simulink model "Import_IMU"  (R2023b)
settings: Solver=FixedStepDiscrete  StartTime=0.0  StopTime=inf  FixedStep=0.003  RelTol=1e-3
InitFcn:
  | run('dual_leg_init.m');
values from neighbouring files (symbols this model uses):
  L1 = single(0.0804)    [dual_leg_init.m]
  L2 = single(0.1200)    [dual_leg_init.m]
  L3 = single(0.1200)    [dual_leg_init.m]
  L4 = single(0.0804)    [dual_leg_init.m]
  L5 = single(0.0700)    [dual_leg_init.m]
undefined symbols (not defined in the file or in its folder): CAL
libraries: ros2lib x14
(part 1 of 2)
settings Model: Creator=root  LastModifiedBy=root
settings OptimizationCC: EnhancedBackFolding=on  PassReuseOutputArgsAs=Individual arguments  ZeroExternalMemoryAtStartup=off  ZeroInternalMemoryAtStartup=off  MaxStackSize=64  OptimizeBlockOrder=speed  DifferentSizesBufferReuse=on  OptimizationCustomize=off  EfficientTunableParamExpr=on
settings DebuggingCC: ParameterTunabilityLossMsg=error
settings HardwareCC: ProdBitPerLong=64  ProdHWDeviceType=Intel->x86-64 (Linux 64)
settings SFSimCC: MATLABDynamicMemAlloc=off
settings RTWCC: Description=Embedded Coder  SystemTargetFile=ert.tlc  HardwareBoard=Robot Operating System 2 (ROS 2)  TLCOptions="-aInlineSetEventsForThisBaseRateFcn=TLC_FALSE -aSuppressMultiTaskScheduler=TLC_FALSE  -aRateBasedStepFcn=0"  TemplateMakefile=ert_default_tmf  Toolchain=Colcon Tools  TargetLang=C++
settings CodeAppCC: ForceParamTrailComments=on  IgnoreCustomStorageClasses=off  OperatorAnnotations=on  SimulinkDataObjDesc=on  SFDataObjDesc=on  InsertBlockDesc=on
settings ERTTargetCC: CodeInterfacePackaging=C++ class  SupportContinuousTime=on  RootIOFormat=Structure reference

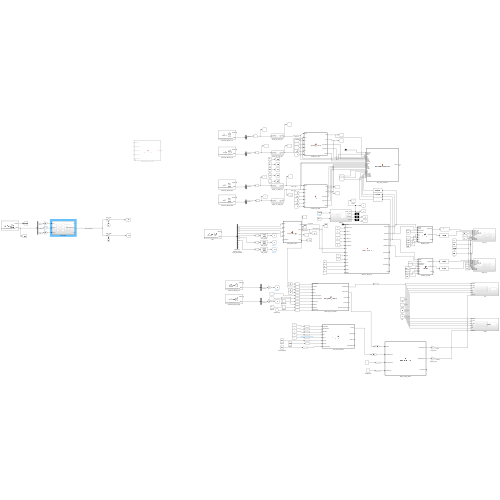
[thumbnail: Simulink's stored preview of the top-level diagram]
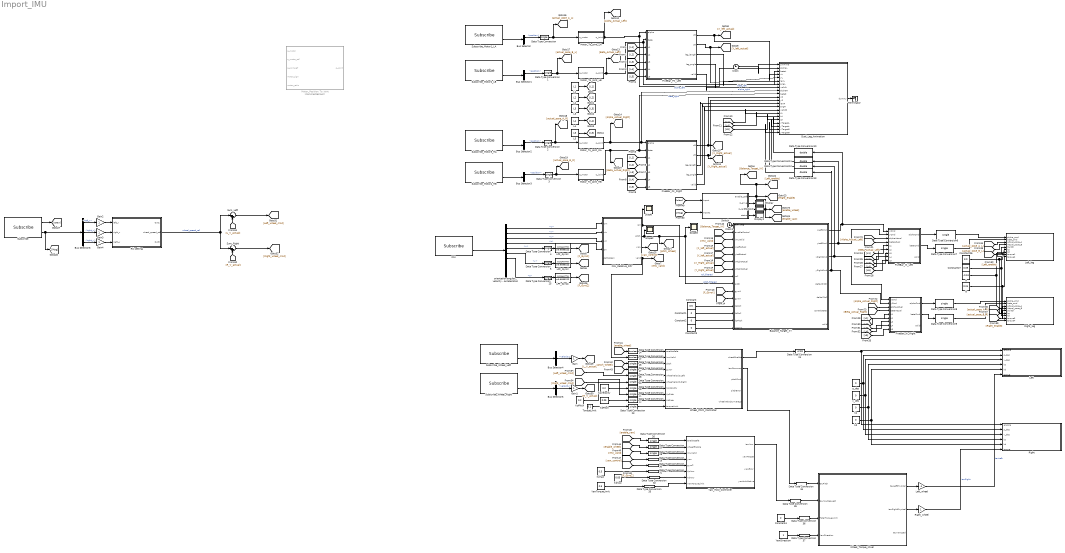
== system Import_IMU ==
  A : Constant  Value=-0.24
  B : Constant  Value=0.24
  Balance_Target_XY : MATLAB Function  TreatAsAtomicUnit=on
  Bus Selector{,1..5} (6 alike) : BusSelector  OutputSignals=position,velocity,torque
  Bus Selector6 : BusSelector  OutputSignals=left_x,right_x,right_y
  Clock : Clock
  Clock1 : Clock
  Constant : Constant  Value=0.5
  Constant1 : Constant  Value=0
  Constant2 : Constant  Value=0
  Constant26 : Constant  Value=3.0
  Constant27 : Constant  Value=0.09
  Constant3 : Constant  Value=0
  Constant4 : Constant  Value=2
  Data Type Conversion{,1..9,16..23,25..37} (31 alike) : DataTypeConversion  OutDataTypeStr=single  SaturateOnIntegerOverflow=off  RndMeth=Floor
  Data Type Conversion{10..13} (4 alike) : DataTypeConversion  OutDataTypeStr=double  SaturateOnIntegerOverflow=off  RndMeth=Floor
  Data Type Conversion14 : DataTypeConversion  OutDataTypeStr=boolean  SaturateOnIntegerOverflow=off  RndMeth=Floor
  Data Type Conversion15 : DataTypeConversion  OutDataTypeStr=boolean  SaturateOnIntegerOverflow=off  RndMeth=Floor
  Data Type Conversion24 : DataTypeConversion  OutDataTypeStr=uint8  SaturateOnIntegerOverflow=off  RndMeth=Floor
  Display : Display
  Display1 : Display
  Display2 : Display
  Dual_Leg_Animation : MATLAB Function  TreatAsAtomicUnit=on
  FiveBar_FK_Left : MATLAB Function  TreatAsAtomicUnit=on
  FiveBar_FK_Right : MATLAB Function  TreatAsAtomicUnit=on
  FiveBar_IK_Left : MATLAB Function  TreatAsAtomicUnit=on
  FiveBar_IK_Right : MATLAB Function  TreatAsAtomicUnit=on
  Gain : Gain
  Gain1 : Gain
  Gain2 : Gain  OutDataTypeStr=single
  Gain3 : Gain  OutDataTypeStr=single
  Gain4 : Gain  OutDataTypeStr=single
  IMU : ros2lib/Subscribe  topicSource=Select from ROS network  topic=/ecat/sn1966149/app1/read  messageType=sensor_msgs/Imu  sampleTime=-1  QOSHistory=Keep last  QOSDepth=1  QOSReliability=Best effort  QOSDurability=Volatile
  IMU_Relative_RPY : MATLAB Function  TreatAsAtomicUnit=on
  KdPitch : Constant  Value=0.05
  KdYaw : Constant  Value=0.05
  KpPitch : Constant  Value=0.2
  KpVelocity : Constant  Value=0.2
  KpYaw : Constant  Value=0.5
  L1 : Constant  Value=L1
  L2 : Constant  Value=L2
  L3 : Constant  Value=L3
  L4 : Constant  Value=L4
  L5 : Constant  Value=L5
  LPF_GyroX : DiscreteTransferFcn  Numerator=[0.3140778]  Denominator=[1 -0.6859222]
  LPF_GyroY : DiscreteTransferFcn  Numerator=[0.3140778]  Denominator=[1 -0.6859222]
  LPF_GyroZ : DiscreteTransferFcn  Numerator=[0.3140778]  Denominator=[1 -0.6859222]
  Left : Subsystem
  Left_leg : Subsystem
  Left_wheel : Gain  Gain=-1
  Motor_Position_To_Joint : MATLAB Function  Commented=on  TreatAsAtomicUnit=on
  Motor_To_Joint_LA : Subsystem
  Motor_To_Joint_LB : Subsystem
  Motor_To_Joint_RA : Subsystem
  Motor_To_Joint_RB : Subsystem
  RC setting : Subsystem
  Right : Subsystem
  Right_leg : Subsystem
  Right_wheel : Gain
  Scope : Scope
  Scope2 : Scope
  Scope3 : Scope
  Subscribe : ros2lib/Subscribe  topicSource=Select from ROS network  topic=/ecat/sn2228252/app1/read  messageType=custom_msgs/ReadDJIRC  sampleTime=-1  QOSHistory=Keep last  QOSDepth=1  QOSReliability=Best effort  QOSDurability=Volatile
  Subscribe_Motor1_LA : ros2lib/Subscribe  topicSource=Select from ROS network  topic=/ecat/sn2228252/app2/read  messageType=custom_msgs/ReadDmMotor  sampleTime=-1  QOSHistory=Keep last  QOSDepth=1  QOSReliability=Best effort  QOSDurability=Volatile
  Subscribe_Motor2_LB : ros2lib/Subscribe  topicSource=Select from ROS network  topic=/ecat/sn2228252/app3/read  messageType=custom_msgs/ReadDmMotor  sampleTime=-1  QOSHistory=Keep last  QOSDepth=1  QOSReliability=Best effort  QOSDurability=Volatile
  Subscribe_Motor3_RA : ros2lib/Subscribe  topicSource=Select from ROS network  topic=/ecat/sn2228252/app5/read  messageType=custom_msgs/ReadDmMotor  sampleTime=-1  QOSHistory=Keep last  QOSDepth=1  QOSReliability=Best effort  QOSDurability=Volatile
  Subscribe_Motor4_RB : ros2lib/Subscribe  topicSource=Select from ROS network  topic=/ecat/sn2228252/app6/read  messageType=custom_msgs/ReadDmMotor  sampleTime=-1  QOSHistory=Keep last  QOSDepth=1  QOSReliability=Best effort  QOSDurability=Volatile
  Subscribe_Wheel_Left : ros2lib/Subscribe  topicSource=Select from ROS network  topic=/ecat/sn2228252/app4/read  messageType=custom_msgs/ReadDmMotor  sampleTime=-1  QOSHistory=Keep last  QOSDepth=1  QOSReliability=Best effort  QOSDurability=Volatile
  Subscribe_Wheel_Right : ros2lib/Subscribe  topicSource=Select from ROS network  topic=/ecat/sn2228252/app7/read  messageType=custom_msgs/ReadDmMotor  sampleTime=-1  QOSHistory=Keep last  QOSDepth=1  QOSReliability=Best effort  QOSDurability=Volatile
  Sum_Left : Sum  Inputs=|-+
  Sum_Right : Sum  Inputs=|-+
  Switch : Subsystem
  Terminator : Terminator
  TorqueLimit : Constant  Value=0.1
  Wheel_Pitch_Controller : MATLAB Function  TreatAsAtomicUnit=on
  Wheel_Torque_Mixer : MATLAB Function  TreatAsAtomicUnit=on
  YawDirection : Constant
  YawTorqueLimit : Constant  Value=0.5
  Yaw_Hold_Controller : MATLAB Function  TreatAsAtomicUnit=on
  kd : Constant  Value=0  OutDataTypeStr=single
  kp : Constant  Value=0  OutDataTypeStr=single
  orientation angular_velocity linear_acceleration : BusSelector  OutputSignals=orientation.w,orientation.x,orientation.y,orientation.z,angular_velocity.x,angular_velocity.y,angular_velocity.z,linear_acceleration.x,linear_acceleration.y,linear_acceleration.z
  p_des : Constant  Value=0  OutDataTypeStr=single
  v_des : Constant  Value=0  OutDataTypeStr=single
  wires:
  Subscribe_Motor1_LA/2 -> Bus Selector/1
  Subscribe_Motor2_LB/2 -> Bus Selector1/1
  Subscribe_Motor3_RA/2 -> Bus Selector2/1
  Subscribe_Motor4_RB/2 -> Bus Selector3/1
  Bus Selector/1 -> Data Type Conversion/1  "<position>"
  Bus Selector1/1 -> Data Type Conversion1/1  "<position>"
  Bus Selector2/1 -> Data Type Conversion2/1  "<position>"
  Bus Selector3/1 -> Data Type Conversion3/1  "<position>"
  Motor_To_Joint_LA/1(q_joint) -> Dual_Leg_Animation/2(alphaL), FiveBar_FK_Left/1(alpha), [Alpha_Actual_Left]  "alpha_left"
  Motor_To_Joint_LB/1(q_joint) -> [Beta_Actual_Left], Dual_Leg_Animation/3(betaL), FiveBar_FK_Left/2(beta)  "beta_left"
  Motor_To_Joint_RA/1(q_joint) -> [Alpha_Actual_Right], Dual_Leg_Animation/9(alphaR), FiveBar_FK_Right/1(alpha)  "alpha_right"
  Motor_To_Joint_RB/1(q_joint) -> [Beta_Actual_Right], Dual_Leg_Animation/10(betaR), FiveBar_FK_Right/2(beta)  "beta_right"
  L1/1 -> [L1]
  L2/1 -> [L2]
  L3/1 -> [L3]
  L4/1 -> [L4]
  L5/1 -> [L5]
  [L1] -> FiveBar_FK_Left/3(L1)
  [L2] -> FiveBar_FK_Left/4(L2)
  [L3] -> FiveBar_FK_Left/5(L3)
  [L4] -> FiveBar_FK_Left/6(L4)
  [L5] -> FiveBar_FK_Left/7(L5)
  [L1] -> FiveBar_FK_Right/3(L1)
  [L2] -> FiveBar_FK_Right/4(L2)
  [L3] -> FiveBar_FK_Right/5(L3)
  [L4] -> FiveBar_FK_Right/6(L4)
  [L5] -> FiveBar_FK_Right/7(L5)
  Data Type Conversion/1 -> [actual_pose_A_L], Motor_To_Joint_LA/1(q_motor)
  Data Type Conversion1/1 -> [actual_pose_B_L], Motor_To_Joint_LB/1(q_motor)
  Data Type Conversion2/1 -> [actual_pose_A_R], Motor_To_Joint_RA/1(q_motor)
  Data Type Conversion3/1 -> [actual_pose_B_R], Motor_To_Joint_RB/1(q_motor)
  Clock/1 -> Dual_Leg_Animation/1(simTime)
  FiveBar_FK_Left/1(xB) -> [X_left_actual], Dual_Leg_Animation/4(xL)
  FiveBar_FK_Left/2(yB) -> [Y_left_actual], Dual_Leg_Animation/5(yL)
  FiveBar_FK_Left/3(leg_length) -> Dual_Leg_Animation/6(lenL)
  FiveBar_FK_Left/4(leg_angle) -> Dual_Leg_Animation/7(angL)
  FiveBar_FK_Left/5(valid) -> Dual_Leg_Animation/8(validL)
  FiveBar_FK_Right/1(xB) -> Dual_Leg_Animation/11(xR), [X_Right_actual]
  FiveBar_FK_Right/2(yB) -> [Y_Right_actual], Dual_Leg_Animation/12(yR)
  FiveBar_FK_Right/3(leg_length) -> Dual_Leg_Animation/13(lenR)
  FiveBar_FK_Right/4(leg_angle) -> Dual_Leg_Animation/14(angR)
  FiveBar_FK_Right/5(valid) -> Dual_Leg_Animation/15(validR)
  [L1] -> Dual_Leg_Animation/16(L1)
  [L4] -> Dual_Leg_Animation/17(L4)
  [L5] -> Dual_Leg_Animation/18(L5)
  Dual_Leg_Animation/1(dummy) -> Terminator/1
  IMU/2 -> orientation angular_velocity linear_acceleration/1
  orientation angular_velocity linear_acceleration/1 -> IMU_Relative_RPY/1(wIn)  "<w>"
  orientation angular_velocity linear_acceleration/2 -> IMU_Relative_RPY/2(xIn)  "<x>"
  orientation angular_velocity linear_acceleration/3 -> IMU_Relative_RPY/3(yIn)  "<y>"
  orientation angular_velocity linear_acceleration/4 -> IMU_Relative_RPY/4(zIn)  "<z>"
  IMU_Relative_RPY/1(roll) -> Balance_Target_XY/8(roll), Scope/1  "roll_filtered"
  IMU_Relative_RPY/2(pitch) -> [pitch_Wheel], Scope3/1, Balance_Target_XY/9(pitch), Scope2/1  "pitch_filtered"
  orientation angular_velocity linear_acceleration/5 -> Data Type Conversion4/1  "<x>"
  orientation angular_velocity linear_acceleration/6 -> Data Type Conversion5/1  "<y>"
  Data Type Conversion4/1 -> LPF_GyroX/1
  Data Type Conversion5/1 -> LPF_GyroY/1
  LPF_GyroX/1 -> [F_GyroX]
  LPF_GyroY/1 -> [F_GyroY]
  [F_GyroX] -> Balance_Target_XY/10(gyroX)
  [F_GyroY] -> Balance_Target_XY/11(gyroY)
  Clock1/1 -> Balance_Target_XY/1(simTime)
  [IMU_valid] -> Balance_Target_XY/3(imuValid)
  [X_left_actual] -> Balance_Target_XY/4(xLeftActual)
  [Y_left_actual] -> Balance_Target_XY/5(yLeftActual)
  [X_Right_actual] -> Balance_Target_XY/6(xRightActual)
  [Y_Right_actual] -> Balance_Target_XY/7(yRightActual)
  Constant/1 -> Balance_Target_XY/12(kpRoll)
  Constant1/1 -> Balance_Target_XY/13(kdRoll)
  Constant2/1 -> Balance_Target_XY/14(kpPitch)
  Constant3/1 -> Balance_Target_XY/15(kdPitch)
  Balance_Target_XY/1(xLeftCmd) -> Data Type Conversion10/1, FiveBar_IK_Left/1(xCmd)
  Balance_Target_XY/2(yLeftCmd) -> Data Type Conversion11/1, FiveBar_IK_Left/2(yCmd)
  Balance_Target_XY/3(xRightCmd) -> Data Type Conversion12/1, FiveBar_IK_Right/1(xCmd)
  Balance_Target_XY/4(yRightCmd) -> FiveBar_IK_Right/2(yCmd), Data Type Conversion13/1
  [Alpha_Actual_Left] -> FiveBar_IK_Left/3(alphaActual)
  [Beta_Actual_Left] -> FiveBar_IK_Left/4(betaActual)
  [Alpha_Actual_Right] -> FiveBar_IK_Right/3(alphaActual)
  [Beta_Actual_Right] -> FiveBar_IK_Right/4(betaActual)
  [L1] -> FiveBar_IK_Left/5(L1)
  [L2] -> FiveBar_IK_Left/6(L2)
  [L3] -> FiveBar_IK_Left/7(L3)
  [L4] -> FiveBar_IK_Left/8(L4)
  [L5] -> FiveBar_IK_Left/9(L5)
  [L1] -> FiveBar_IK_Right/5(L1)
  [L2] -> FiveBar_IK_Right/6(L2)
  [L3] -> FiveBar_IK_Right/7(L3)
  [L4] -> FiveBar_IK_Right/8(L4)
  [L5] -> FiveBar_IK_Right/9(L5)
  IMU_Relative_RPY/4(valid) -> [IMU_valid], Data Type Conversion15/1
  FiveBar_IK_Left/1(alphaCmd) -> Data Type Conversion6/1
  Data Type Conversion6/1 -> Left_leg/1(alpha_cmd)
  FiveBar_IK_Left/2(betaCmd) -> Data Type Conversion7/1
  Data Type Conversion7/1 -> Left_leg/2(beta_cmd)
  FiveBar_IK_Right/1(alphaCmd) -> Data Type Conversion8/1
  Data Type Conversion8/1 -> Right_leg/1(alpha_cmd)
  FiveBar_IK_Right/2(betaCmd) -> Data Type Conversion9/1
  Data Type Conversion9/1 -> Right_leg/2(beta_cmd)
  [actual_pose_A_L] -> Left_leg/3(Actual_pose_A)
  [actual_pose_B_L] -> Left_leg/4(Actual_pose_B)
  [actual_pose_A_R] -> Right_leg/3(Actual_pose_A)
  [actual_pose_B_R] -> Right_leg/4(Actual_pose_B)
  [Right_enable] -> Right_leg/5(Switch)
  [Left_enable] -> Left_leg/5(Switch)
  Switch/1(enable_safe) -> [enable_yaw], [enable_wheel], [Right_enable], [Left_enable], [Balance_Target_XY]
  [Balance_Target_XY] -> Balance_Target_XY/2(enableControl)
  Switch/2(rc_alive) -> Display/1
  Switch/3(rc_ready) -> Display1/1
  Switch/4(status) -> Display2/1
  Constant26/1 -> Right_leg/6(kp), Left_leg/6(kp)
  Constant27/1 -> Right_leg/7(kd), Left_leg/7(kd)
  A/1 -> Left_leg/8(torque1), Right_leg/9(torque4)
  B/1 -> Right_leg/8(torque3), Left_leg/9(torque2)
  Data Type Conversion10/1 -> Dual_Leg_Animation/19(xTargetL)
  Data Type Conversion11/1 -> Dual_Leg_Animation/20(yTargetL)
  Data Type Conversion12/1 -> Dual_Leg_Animation/21(xTargetR)
  Data Type Conversion13/1 -> Dual_Leg_Animation/22(yTargetR)
  Subscribe_Wheel_Left/2 -> Bus Selector4/1
  Subscribe_Wheel_Right/2 -> Bus Selector5/1
  Bus Selector4/2 -> Gain/1  "<velocity>"
  Bus Selector5/2 -> Gain1/1  "<velocity>"
  Data Type Conversion14/1 -> Wheel_Pitch_Controller/1(enableSafe)
  Data Type Conversion15/1 -> Wheel_Pitch_Controller/2(imuValid)
  Data Type Conversion16/1 -> Wheel_Pitch_Controller/3(pitch)
  Data Type Conversion17/1 -> Wheel_Pitch_Controller/4(gyroY)
  Data Type Conversion18/1 -> Wheel_Pitch_Controller/5(wheelVelocityLeft)
  Data Type Conversion20/1 -> Wheel_Pitch_Controller/6(wheelVelocityRight)
  Data Type Conversion19/1 -> Wheel_Pitch_Controller/7(KpVelocity)
  Data Type Conversion21/1 -> Wheel_Pitch_Controller/8(KpPitch)
  Data Type Conversion22/1 -> Wheel_Pitch_Controller/9(KdPitch)
  Data Type Conversion23/1 -> Wheel_Pitch_Controller/10(torqueLimit)
  [enable_wheel] -> Data Type Conversion14/1
  [pitch_Wheel] -> Data Type Conversion16/1
  [F_GyroY] -> Data Type Conversion17/1
  KpVelocity/1 -> Data Type Conversion19/1
  KpPitch/1 -> Data Type Conversion21/1
  KdPitch/1 -> Data Type Conversion22/1
  TorqueLimit/1 -> Data Type Conversion23/1
  Wheel_Pitch_Controller/2(tauCommon) -> Data Type Conversion34/1
  Wheel_Pitch_Controller/1(wheelEnable) -> Data Type Conversion24/1
  Data Type Conversion24/1 -> Right/1(enable), Left/1(enable)
  p_des/1 -> Right/2(p_des), Left/2(p_des)
  v_des/1 -> Left/3(v_des), Right/3(v_des)
  kp/1 -> Right/4(kp), Left/4(kp)
  kd/1 -> Right/5(kd), Left/5(kd)
  orientation angular_velocity linear_acceleration/7 -> Data Type Conversion25/1  "<z>"
  Data Type Conversion25/1 -> LPF_GyroZ/1
  [enable_wheel] -> Data Type Conversion27/1
  [enable_yaw] -> Data Type Conversion26/1
  [IMU_valid] -> Data Type Conversion28/1
  IMU_Relative_RPY/3(yaw) -> [yaw_control]
  [yaw_control] -> Data Type Conversion29/1
  LPF_GyroZ/1 -> [F_GyroZ]
  [F_GyroZ] -> Data Type Conversion30/1
  YawTorqueLimit/1 -> Data Type Conversion33/1
  KdYaw/1 -> Data Type Conversion32/1
  KpYaw/1 -> Data Type Conversion31/1
  YawDirection/1 -> Data Type Conversion37/1
  Yaw_Hold_Controller/1(tauYaw) -> Data Type Conversion35/1
  Wheel_Torque_Mixer/1(tauLeftPhysical) -> Left_wheel/1
  Left_wheel/1 -> Left/6(torque)  "tauLeft"
  Wheel_Torque_Mixer/2(tauRightPhysical) -> Right_wheel/1
  Right_wheel/1 -> Right/6(torque)  "tauRight"
  Constant4/1 -> Data Type Conversion36/1
  Data Type Conversion26/1 -> Yaw_Hold_Controller/1(enableSafe)
  Data Type Conversion27/1 -> Yaw_Hold_Controller/2(wheelEnable)
  Data Type Conversion28/1 -> Yaw_Hold_Controller/3(imuValid)
  Data Type Conversion29/1 -> Yaw_Hold_Controller/4(yaw)
  Data Type Conversion30/1 -> Yaw_Hold_Controller/5(gyroZ)
  Data Type Conversion31/1 -> Yaw_Hold_Controller/6(KpYaw)
  Data Type Conversion32/1 -> Yaw_Hold_Controller/7(KdYaw)
  Data Type Conversion33/1 -> Yaw_Hold_Controller/8(YawTorqueLimit)
  Data Type Conversion34/1 -> Wheel_Torque_Mixer/1(tauPitch)
  Data Type Conversion35/1 -> Wheel_Torque_Mixer/2(tauYawRequest)
  Data Type Conversion36/1 -> Wheel_Torque_Mixer/3(TotalTorqueLimit)
  Data Type Conversion37/1 -> Wheel_Torque_Mixer/4(YawDirection)
  Subscribe/1 -> [IsNew]
  Subscribe/2 -> [Msg], Bus Selector6/1
  [IsNew] -> Switch/1(Inport)
  [Msg] -> Switch/2(Inport1)
  Bus Selector6/1 -> Gain2/1  "<left_x>"
  Bus Selector6/2 -> Gain3/1  "<right_x>"
  Bus Selector6/3 -> Gain4/1  "<right_y>"
  Gain3/1 -> RC setting/2(right_x)
  Gain2/1 -> RC setting/1(left_x)
  Gain4/1 -> RC setting/3(right_y)
  RC setting/2(wheel_speed_ref) -> Sum_Right/1, Sum_Left/1  "wheel_speed_ref"
  Gain/1 -> [L_V_actual]
  Gain1/1 -> [R_V_actual]
  [L_V_actual] -> Sum_Left/2
  [R_V_actual] -> Sum_Right/2
  Sum_Left/1 -> [Left_wheel_cmd]
  Sum_Right/1 -> [Right_wheel_cmd]
  [Left_wheel_cmd] -> Data Type Conversion18/1
  [Right_wheel_cmd] -> Data Type Conversion20/1

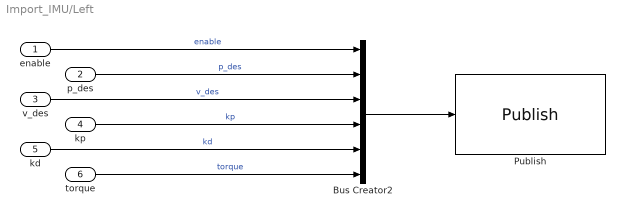
== system Import_IMU/Left ==
  enable : Inport
  p_des : Inport  Port=2
  v_des : Inport  Port=3
  kp : Inport  Port=4
  kd : Inport  Port=5
  torque : Inport  Port=6
  Bus Creator2 : BusCreator  Inputs=6  OutDataTypeStr=Bus: SL_Bus_custom_msgs_WriteDmMotorMITControl  NonVirtualBus=on
  Publish : ros2lib/Publish  topicSource=Select from ROS network  topic=/ecat/sn2228252/app4/write  messageType=custom_msgs/WriteDmMotorMITControl  QOSHistory=Keep last  QOSDepth=1  QOSReliability=Best effort  QOSDurability=Volatile
  wires:
  enable/1 -> Bus Creator2/1  "enable"
  Bus Creator2/1 -> Publish/1
  p_des/1 -> Bus Creator2/2  "p_des"
  v_des/1 -> Bus Creator2/3  "v_des"
  kp/1 -> Bus Creator2/4  "kp"
  kd/1 -> Bus Creator2/5  "kd"
  torque/1 -> Bus Creator2/6  "torque"

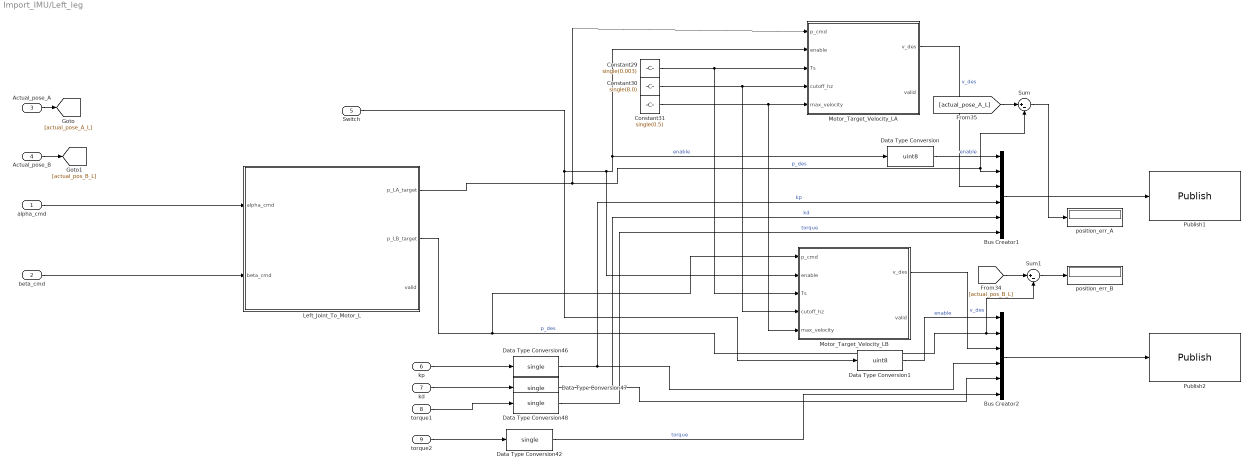
== system Import_IMU/Left_leg ==
  alpha_cmd : Inport
  beta_cmd : Inport  Port=2
  Actual_pose_A : Inport  Port=3
  Actual_pose_B : Inport  Port=4
  Switch : Inport  Port=5
  kp : Inport  Port=6
  kd : Inport  Port=7
  torque1 : Inport  Port=8
  torque2 : Inport  Port=9
  Bus Creator1 : BusCreator  Inputs=6  OutDataTypeStr=Bus: SL_Bus_custom_msgs_WriteDmMotorMITControl  NonVirtualBus=on
  Bus Creator2 : BusCreator  Inputs=6  OutDataTypeStr=Bus: SL_Bus_custom_msgs_WriteDmMotorMITControl  NonVirtualBus=on
  Constant29 : Constant  Value=single(0.003)
  Constant30 : Constant  Value=single(8.0)
  Constant31 : Constant  Value=single(0.5)
  Data Type Conversion : DataTypeConversion  OutDataTypeStr=uint8  SaturateOnIntegerOverflow=off  RndMeth=Floor
  Data Type Conversion1 : DataTypeConversion  OutDataTypeStr=uint8  SaturateOnIntegerOverflow=off  RndMeth=Floor
  Data Type Conversion{42,46..48} (4 alike) : DataTypeConversion  OutDataTypeStr=single  SaturateOnIntegerOverflow=off  RndMeth=Floor
  Left_Joint_To_Motor_L : MATLAB Function  TreatAsAtomicUnit=on
  Motor_Target_Velocity_LA : MATLAB Function  TreatAsAtomicUnit=on
  Motor_Target_Velocity_LB : MATLAB Function  TreatAsAtomicUnit=on
  Publish1 : ros2lib/Publish  topicSource=Select from ROS network  topic=/ecat/sn2228252/app2/write  messageType=custom_msgs/WriteDmMotorMITControl  QOSHistory=Keep last  QOSDepth=1  QOSReliability=Best effort  QOSDurability=Volatile
  Publish2 : ros2lib/Publish  topicSource=Select from ROS network  topic=/ecat/sn2228252/app3/write  messageType=custom_msgs/WriteDmMotorMITControl  QOSHistory=Keep last  QOSDepth=1  QOSReliability=Best effort  QOSDurability=Volatile
  Sum : Sum  Inputs=|+-
  Sum1 : Sum  Inputs=|+-
  position_err_A : Display
  position_err_B : Display
  wires:
  Motor_Target_Velocity_LA/1(v_des) -> Bus Creator1/3  "v_des"
  kp/1 -> Data Type Conversion46/1
  torque1/1 -> Data Type Conversion48/1
  Constant30/1 -> Motor_Target_Velocity_LB/4(cutoff_hz), Motor_Target_Velocity_LA/4(cutoff_hz)
  Data Type Conversion47/1 -> Bus Creator1/5, Bus Creator2/5  "kd"
  Switch/1 -> Data Type Conversion1/1, Motor_Target_Velocity_LB/2(enable), Motor_Target_Velocity_LA/2(enable), Data Type Conversion/1  "enable"
  Sum/1 -> position_err_A/1
  Data Type Conversion48/1 -> Bus Creator1/6  "torque"
  Sum1/1 -> position_err_B/1
  Data Type Conversion46/1 -> Bus Creator1/4, Bus Creator2/4  "kp"
  Constant29/1 -> Motor_Target_Velocity_LB/3(Ts), Motor_Target_Velocity_LA/3(Ts)
  [actual_pos_B_L] -> Sum1/1
  Motor_Target_Velocity_LB/1(v_des) -> Bus Creator2/3  "v_des"
  Left_Joint_To_Motor_L/1(p_LA_target) -> Motor_Target_Velocity_LA/1(p_cmd), Sum/2, Bus Creator1/2  "p_des"
  Constant31/1 -> Motor_Target_Velocity_LB/5(max_velocity), Motor_Target_Velocity_LA/5(max_velocity)
  kd/1 -> Data Type Conversion47/1
  [actual_pose_A_L] -> Sum/1
  Bus Creator2/1 -> Publish2/1
  Data Type Conversion42/1 -> Bus Creator2/6  "torque"
  Left_Joint_To_Motor_L/2(p_LB_target) -> Motor_Target_Velocity_LB/1(p_cmd), Sum1/2, Bus Creator2/2  "p_des"
  Bus Creator1/1 -> Publish1/1
  alpha_cmd/1 -> Left_Joint_To_Motor_L/1(alpha_cmd)
  beta_cmd/1 -> Left_Joint_To_Motor_L/2(beta_cmd)
  torque2/1 -> Data Type Conversion42/1
  Actual_pose_A/1 -> [actual_pose_A_L]
  Actual_pose_B/1 -> [actual_pos_B_L]
  Data Type Conversion/1 -> Bus Creator1/1  "enable"
  Data Type Conversion1/1 -> Bus Creator2/1  "enable"

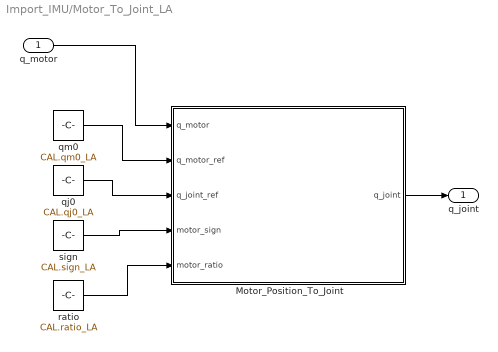
== system Import_IMU/Motor_To_Joint_LA ==
  q_motor : Inport
  Motor_Position_To_Joint : MATLAB Function  TreatAsAtomicUnit=on
  qj0 : Constant  Value=CAL.qj0_LA
  qm0 : Constant  Value=CAL.qm0_LA
  ratio : Constant  Value=CAL.ratio_LA
  sign : Constant  Value=CAL.sign_LA
  q_joint : Outport
  wires:
  q_motor/1 -> Motor_Position_To_Joint/1(q_motor)
  qm0/1 -> Motor_Position_To_Joint/2(q_motor_ref)
  qj0/1 -> Motor_Position_To_Joint/3(q_joint_ref)
  sign/1 -> Motor_Position_To_Joint/4(motor_sign)
  ratio/1 -> Motor_Position_To_Joint/5(motor_ratio)
  Motor_Position_To_Joint/1(q_joint) -> q_joint/1

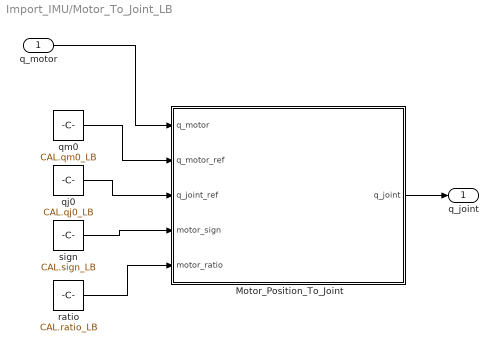
== system Import_IMU/Motor_To_Joint_LB ==
  q_motor : Inport
  Motor_Position_To_Joint : MATLAB Function  TreatAsAtomicUnit=on
  qj0 : Constant  Value=CAL.qj0_LB
  qm0 : Constant  Value=CAL.qm0_LB
  ratio : Constant  Value=CAL.ratio_LB
  sign : Constant  Value=CAL.sign_LB
  q_joint : Outport
  wires:
  q_motor/1 -> Motor_Position_To_Joint/1(q_motor)
  qm0/1 -> Motor_Position_To_Joint/2(q_motor_ref)
  qj0/1 -> Motor_Position_To_Joint/3(q_joint_ref)
  sign/1 -> Motor_Position_To_Joint/4(motor_sign)
  ratio/1 -> Motor_Position_To_Joint/5(motor_ratio)
  Motor_Position_To_Joint/1(q_joint) -> q_joint/1

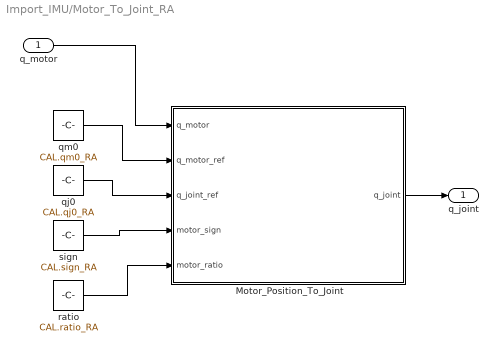
== system Import_IMU/Motor_To_Joint_RA ==
  q_motor : Inport
  Motor_Position_To_Joint : MATLAB Function  TreatAsAtomicUnit=on
  qj0 : Constant  Value=CAL.qj0_RA
  qm0 : Constant  Value=CAL.qm0_RA
  ratio : Constant  Value=CAL.ratio_RA
  sign : Constant  Value=CAL.sign_RA
  q_joint : Outport
  wires:
  q_motor/1 -> Motor_Position_To_Joint/1(q_motor)
  qm0/1 -> Motor_Position_To_Joint/2(q_motor_ref)
  qj0/1 -> Motor_Position_To_Joint/3(q_joint_ref)
  sign/1 -> Motor_Position_To_Joint/4(motor_sign)
  ratio/1 -> Motor_Position_To_Joint/5(motor_ratio)
  Motor_Position_To_Joint/1(q_joint) -> q_joint/1

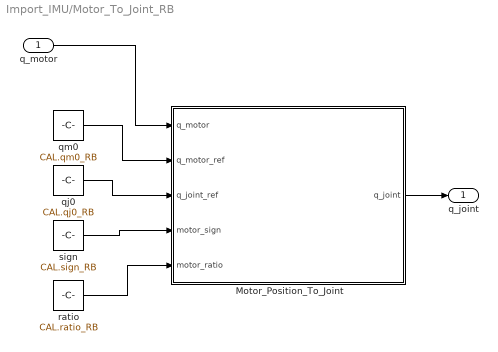
== system Import_IMU/Motor_To_Joint_RB ==
  q_motor : Inport
  Motor_Position_To_Joint : MATLAB Function  TreatAsAtomicUnit=on
  qj0 : Constant  Value=CAL.qj0_RB
  qm0 : Constant  Value=CAL.qm0_RB
  ratio : Constant  Value=CAL.ratio_RB
  sign : Constant  Value=CAL.sign_RB
  q_joint : Outport
  wires:
  q_motor/1 -> Motor_Position_To_Joint/1(q_motor)
  qm0/1 -> Motor_Position_To_Joint/2(q_motor_ref)
  qj0/1 -> Motor_Position_To_Joint/3(q_joint_ref)
  sign/1 -> Motor_Position_To_Joint/4(motor_sign)
  ratio/1 -> Motor_Position_To_Joint/5(motor_ratio)
  Motor_Position_To_Joint/1(q_joint) -> q_joint/1

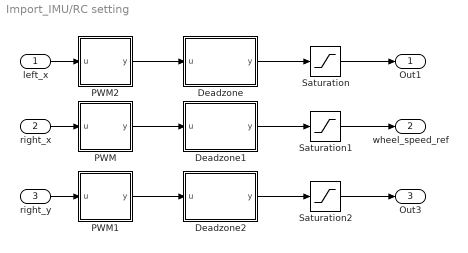
== system Import_IMU/RC setting ==
  left_x : Inport
  right_x : Inport  Port=2
  right_y : Inport  Port=3
  Deadzone : MATLAB Function  TreatAsAtomicUnit=on
  Deadzone1 : MATLAB Function  TreatAsAtomicUnit=on
  Deadzone2 : MATLAB Function  TreatAsAtomicUnit=on
  PWM : MATLAB Function  TreatAsAtomicUnit=on
  PWM1 : MATLAB Function  TreatAsAtomicUnit=on
  PWM2 : MATLAB Function  TreatAsAtomicUnit=on
  Saturation : Saturate  UpperLimit=1  LowerLimit=-1
  Saturation1 : Saturate  UpperLimit=1  LowerLimit=-1
  Saturation2 : Saturate  UpperLimit=1  LowerLimit=-1
  Out1 : Outport
  wheel_speed_ref : Outport  Port=2
  Out3 : Outport  Port=3
  wires:
  PWM2/1(y) -> Deadzone/1(u)
  Deadzone/1(y) -> Saturation/1
  PWM1/1(y) -> Deadzone2/1(u)
  Deadzone2/1(y) -> Saturation2/1
  PWM/1(y) -> Deadzone1/1(u)
  Deadzone1/1(y) -> Saturation1/1
  left_x/1 -> PWM2/1(u)
  right_x/1 -> PWM/1(u)
  right_y/1 -> PWM1/1(u)
  Saturation/1 -> Out1/1
  Saturation1/1 -> wheel_speed_ref/1
  Saturation2/1 -> Out3/1

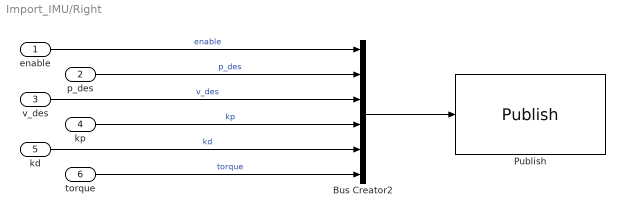
== system Import_IMU/Right ==
  enable : Inport
  p_des : Inport  Port=2
  v_des : Inport  Port=3
  kp : Inport  Port=4
  kd : Inport  Port=5
  torque : Inport  Port=6
  Bus Creator2 : BusCreator  Inputs=6  OutDataTypeStr=Bus: SL_Bus_custom_msgs_WriteDmMotorMITControl  NonVirtualBus=on
  Publish : ros2lib/Publish  topicSource=Select from ROS network  topic=/ecat/sn2228252/app7/write  messageType=custom_msgs/WriteDmMotorMITControl  QOSHistory=Keep last  QOSDepth=1  QOSReliability=Best effort  QOSDurability=Volatile
  wires:
  enable/1 -> Bus Creator2/1  "enable"
  Bus Creator2/1 -> Publish/1
  p_des/1 -> Bus Creator2/2  "p_des"
  v_des/1 -> Bus Creator2/3  "v_des"
  kp/1 -> Bus Creator2/4  "kp"
  kd/1 -> Bus Creator2/5  "kd"
  torque/1 -> Bus Creator2/6  "torque"

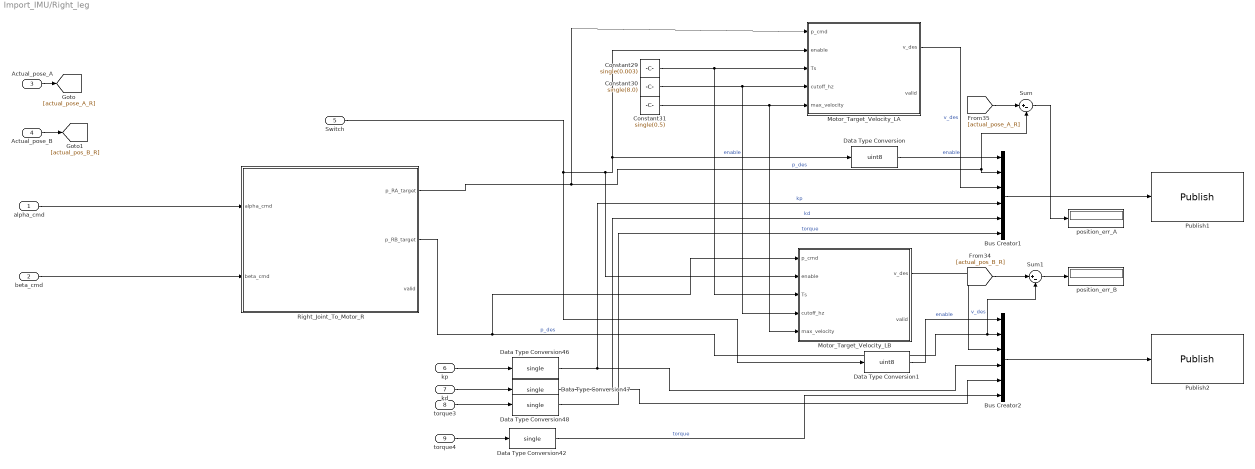
== system Import_IMU/Right_leg ==
  alpha_cmd : Inport
  beta_cmd : Inport  Port=2
  Actual_pose_A : Inport  Port=3
  Actual_pose_B : Inport  Port=4
  Switch : Inport  Port=5
  kp : Inport  Port=6
  kd : Inport  Port=7
  torque3 : Inport  Port=8
  torque4 : Inport  Port=9
  Bus Creator1 : BusCreator  Inputs=6  OutDataTypeStr=Bus: SL_Bus_custom_msgs_WriteDmMotorMITControl  NonVirtualBus=on
  Bus Creator2 : BusCreator  Inputs=6  OutDataTypeStr=Bus: SL_Bus_custom_msgs_WriteDmMotorMITControl  NonVirtualBus=on
  Constant29 : Constant  Value=single(0.003)
  Constant30 : Constant  Value=single(8.0)
  Constant31 : Constant  Value=single(0.5)
  Data Type Conversion : DataTypeConversion  OutDataTypeStr=uint8  SaturateOnIntegerOverflow=off  RndMeth=Floor
  Data Type Conversion1 : DataTypeConversion  OutDataTypeStr=uint8  SaturateOnIntegerOverflow=off  RndMeth=Floor
  Data Type Conversion{42,46..48} (4 alike) : DataTypeConversion  OutDataTypeStr=single  SaturateOnIntegerOverflow=off  RndMeth=Floor
  Motor_Target_Velocity_LA : MATLAB Function  TreatAsAtomicUnit=on
  Motor_Target_Velocity_LB : MATLAB Function  TreatAsAtomicUnit=on
  Publish1 : ros2lib/Publish  topicSource=Select from ROS network  topic=/ecat/sn2228252/app5/write  messageType=custom_msgs/WriteDmMotorMITControl  QOSHistory=Keep last  QOSDepth=1  QOSReliability=Best effort  QOSDurability=Volatile
  Publish2 : ros2lib/Publish  topicSource=Select from ROS network  topic=/ecat/sn2228252/app6/write  messageType=custom_msgs/WriteDmMotorMITControl  QOSHistory=Keep last  QOSDepth=1  QOSReliability=Best effort  QOSDurability=Volatile
  Right_Joint_To_Motor_R : MATLAB Function  TreatAsAtomicUnit=on
  Sum : Sum  Inputs=|+-
  Sum1 : Sum  Inputs=|+-
  position_err_A : Display
  position_err_B : Display
  wires:
  Motor_Target_Velocity_LA/1(v_des) -> Bus Creator1/3  "v_des"
  kp/1 -> Data Type Conversion46/1
  torque3/1 -> Data Type Conversion48/1
  Constant30/1 -> Motor_Target_Velocity_LB/4(cutoff_hz), Motor_Target_Velocity_LA/4(cutoff_hz)
  Data Type Conversion47/1 -> Bus Creator1/5, Bus Creator2/5  "kd"
  Switch/1 -> Data Type Conversion1/1, Motor_Target_Velocity_LB/2(enable), Motor_Target_Velocity_LA/2(enable), Data Type Conversion/1  "enable"
  Sum/1 -> position_err_A/1
  Data Type Conversion48/1 -> Bus Creator1/6  "torque"
  Sum1/1 -> position_err_B/1
  Data Type Conversion46/1 -> Bus Creator1/4, Bus Creator2/4  "kp"
  Constant29/1 -> Motor_Target_Velocity_LB/3(Ts), Motor_Target_Velocity_LA/3(Ts)
  [actual_pos_B_R] -> Sum1/1
  Motor_Target_Velocity_LB/1(v_des) -> Bus Creator2/3  "v_des"
  Right_Joint_To_Motor_R/1(p_RA_target) -> Motor_Target_Velocity_LA/1(p_cmd), Sum/2, Bus Creator1/2  "p_des"
  Constant31/1 -> Motor_Target_Velocity_LB/5(max_velocity), Motor_Target_Velocity_LA/5(max_velocity)
  kd/1 -> Data Type Conversion47/1
  [actual_pose_A_R] -> Sum/1
  Bus Creator2/1 -> Publish2/1
  Data Type Conversion42/1 -> Bus Creator2/6  "torque"
  Right_Joint_To_Motor_R/2(p_RB_target) -> Motor_Target_Velocity_LB/1(p_cmd), Sum1/2, Bus Creator2/2  "p_des"
  Bus Creator1/1 -> Publish1/1
  alpha_cmd/1 -> Right_Joint_To_Motor_R/1(alpha_cmd)
  beta_cmd/1 -> Right_Joint_To_Motor_R/2(beta_cmd)
  torque4/1 -> Data Type Conversion42/1
  Actual_pose_B/1 -> [actual_pos_B_R]
  Actual_pose_A/1 -> [actual_pose_A_R]
  Data Type Conversion/1 -> Bus Creator1/1  "enable"
  Data Type Conversion1/1 -> Bus Creator2/1  "enable"

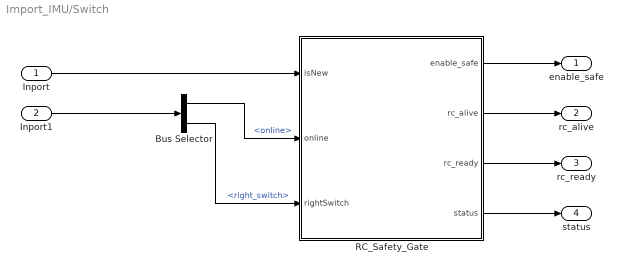
== system Import_IMU/Switch ==
  Inport : Inport
  Inport1 : Inport  Port=2
  Bus Selector : BusSelector  OutputSignals=online,right_switch
  RC_Safety_Gate : MATLAB Function  TreatAsAtomicUnit=on
  enable_safe : Outport  OutDataTypeStr=boolean
  rc_alive : Outport  Port=2
  rc_ready : Outport  Port=3
  status : Outport  Port=4
  wires:
  Bus Selector/1 -> RC_Safety_Gate/2(online)  "<online>"
  Bus Selector/2 -> RC_Safety_Gate/3(rightSwitch)  "<right_switch>"
  RC_Safety_Gate/1(enable_safe) -> enable_safe/1
  RC_Safety_Gate/2(rc_alive) -> rc_alive/1
  RC_Safety_Gate/3(rc_ready) -> rc_ready/1
  RC_Safety_Gate/4(status) -> status/1
  Inport1/1 -> Bus Selector/1
  Inport/1 -> RC_Safety_Gate/1(isNew)

== matlab function Import_IMU/FiveBar_FK_Right ==
  data: alpha input; xB output; beta input; L1 input; L2 input; L3 input; L4 input; L5 input; yB output; leg_length output; leg_angle output; valid output
function [xB, yB, leg_length, leg_angle, valid] = ...
    fivebar_fk_actual(alpha, beta, L1, L2, L3, L4, L5)
%#codegen
%
% 五连杆正运动学
%
% 坐标定义：
% O = (0,0)
% D = (L5,0)
% +x：Alpha电机指向Beta电机
% +y：竖直向下
%
% alpha：O点主动杆角度
% beta ：D点主动杆角度
%
% 输出：
% xB、yB       轮心坐标
% leg_length   基座中点到轮心的虚拟腿长
% leg_angle    虚拟腿相对竖直向下方向的角度
% valid        正运动学是否有效

xB = single(0);
yB = single(0);
leg_length = single(0);
leg_angle = single(0);
valid = false;

%% 主动杆末端A
Ax = L1 * cos(alpha);
Ay = L1 * sin(alpha);

%% 主动杆末端C
Cx = L5 + L4 * cos(beta);
Cy = L4 * sin(beta);

%% A到C的向量
dx = Cx - Ax;
dy = Cy - Ay;

Dac = sqrt(dx*dx + dy*dy);

%% 可达性检查
if Dac < single(1.0e-6)
    return;
end

if Dac > L2 + L3
    return;
end

if Dac < abs(L2 - L3)
    return;
end

%% 两圆交点
a = (L2*L2 - L3*L3 + Dac*Dac) / ...
    (single(2.0) * Dac);

h2 = L2*L2 - a*a;

if h2 < single(-1.0e-7)
    return;
end

if h2 < single(0)
    h2 = single(0);
end

h = sqrt(h2);

ux = dx / Dac;
uy = dy / Dac;

Mx = Ax + a * ux;
My = Ay + a * uy;

%% 两个候选轮心位置
x1 = Mx - h * uy;
y1 = My + h * ux;

x2 = Mx + h * uy;
y2 = My - h * ux;

%% 当前机构中轮心位于更下方，选择y较大的交点
if y1 >= y2
    xB = x1;
    yB = y1;
else
    xB = x2;
    yB = y2;
end

%% 虚拟腿状态
xMid = xB - L5 / single(2.0);

leg_length = sqrt(xMid*xMid + yB*yB);

% 相对于竖直向下方向
leg_angle = atan2(xMid, yB);

valid = true;
end

== matlab function Import_IMU/Dual_Leg_Animation ==
  data: simTime input; dummy output; alphaL input; betaL input; xL input; yL input; lenL input; angL input; validL input; alphaR input; betaR input; xR input; yR input; lenR input; angR input; validR input; L1 input; L4 input; L5 input; xTargetL input; yTargetL input; xTargetR input; yTargetR input
function dummy = dual_leg_animation_block( ...
    simTime, ...
    alphaL, betaL, xL, yL, lenL, angL, validL, ...
    alphaR, betaR, xR, yR, lenR, angR, validR, ...
    L1, L4, L5, ...
    xTargetL, yTargetL, xTargetR, yTargetR)
%#codegen
%
% 双腿五连杆动画调用模块
%
% 新增输入：
%   xTargetL：左腿足端目标x
%   yTargetL：左腿足端目标y
%   xTargetR：右腿足端目标x
%   yTargetR：右腿足端目标y
%
% 该模块仅用于Normal模式动画显示，不参与电机控制。

coder.extrinsic('dual_fivebar_plot');

dual_fivebar_plot( ...
    simTime, ...
    alphaL, betaL, xL, yL, lenL, angL, validL, ...
    alphaR, betaR, xR, yR, lenR, angR, validR, ...
    L1, L4, L5, ...
    xTargetL, yTargetL, xTargetR, yTargetR);

dummy = single(0);

end

== matlab function Import_IMU/IMU_Relative_RPY ==
  data: wIn input; roll output; xIn input; yIn input; zIn input; calibrateIn input; pitch output; yaw output; valid output
function [roll, pitch, yaw, valid] = ...
    imu_relative_rpy(wIn, xIn, yIn, zIn, calibrateIn)
%#codegen
%
% IMU相对姿态解算
%
% 输入：
%   wIn,xIn,yIn,zIn：IMU四元数
%   calibrateIn：零点标定信号，0或1
%
% 输出：
%   roll、pitch、yaw：rad，single
%   valid：logical
%
% 功能：
%   1. 将输入统一转换成single
%   2. 将标定信号统一转换成logical
%   3. 保存零姿态四元数
%   4. 输出相对于零姿态的Roll/Pitch/Yaw

%% 持久变量

persistent q0w q0x q0y q0z
persistent zeroValid
persistent previousCalibrate

if isempty(q0w)

    q0w = single(1.0);
    q0x = single(0.0);
    q0y = single(0.0);
    q0z = single(0.0);

    zeroValid = false;
    previousCalibrate = false;
end

%% 强制统一输入数据类型

w = single(wIn);
x = single(xIn);
y = single(yIn);
z = single(zIn);

% 无论输入是double、uint8还是boolean，都转换成logical
calibrate = calibrateIn ~= 0;

%% 默认输出

roll  = single(0.0);
pitch = single(0.0);
yaw   = single(0.0);
valid = false;

%% 检查当前四元数

inputValid = ...
    isfinite(w) && ...
    isfinite(x) && ...
    isfinite(y) && ...
    isfinite(z);

if ~inputValid
    previousCalibrate = calibrate;
    return;
end

%% 当前四元数归一化

normSquared = ...
    w*w + ...
    x*x + ...
    y*y + ...
    z*z;

if normSquared < single(1.0e-8)
    previousCalibrate = calibrate;
    return;
end

qNorm = sqrt(normSquared);

w = w / qNorm;
x = x / qNorm;
y = y / qNorm;
z = z / qNorm;

%% 检测标定信号上升沿

calibrateRising = ...
    calibrate && ...
    ~previousCalibrate;

%% 首次收到有效IMU数据，或者标定按钮被按下

if calibrateRising || ~zeroValid

    q0w = w;
    q0x = x;
    q0y = y;
    q0z = z;

    zeroValid = true;
end

previousCalibrate = calibrate;

%% 四元数符号连续性处理
%
% q和-q表示同一个姿态。
% 将当前四元数调整到与零点四元数同一半球，
% 防止姿态角突然跳变。

dotValue = ...
    q0w*w + ...
    q0x*x + ...
    q0y*y + ...
    q0z*z;

if dotValue < single(0.0)

    w = -w;
    x = -x;
    y = -y;
    z = -z;
end

%% 计算相对四元数
%
% qRelative = conjugate(qZero) * qCurrent

relativeW = ...
    q0w*w + ...
    q0x*x + ...
    q0y*y + ...
    q0z*z;

relativeX = ...
    q0w*x - ...
    q0x*w - ...
    q0y*z + ...
    q0z*y;

relativeY = ...
    q0w*y + ...
    q0x*z - ...
    q0y*w - ...
    q0z*x;

relativeZ = ...
    q0w*z - ...
    q0x*y + ...
    q0y*x - ...
    q0z*w;

%% 相对四元数再次归一化

relativeNormSquared = ...
    relativeW*relativeW + ...
    relativeX*relativeX + ...
    relativeY*relativeY + ...
    relativeZ*relativeZ;

if relativeNormSquared < single(1.0e-8)
    return;
end

relativeNorm = sqrt(relativeNormSquared);

relativeW = relativeW / relativeNorm;
relativeX = relativeX / relativeNorm;
relativeY = relativeY / relativeNorm;
relativeZ = relativeZ / relativeNorm;

%% 四元数转Roll

sinRoll = single(2.0) * ...
    (relativeW*relativeX + relativeY*relativeZ);

cosRoll = single(1.0) - single(2.0) * ...
    (relativeX*relativeX + relativeY*relativeY);

roll = atan2(sinRoll, cosRoll);

%% 四元数转Pitch

sinPitch = single(2.0) * ...
    (relativeW*relativeY - relativeZ*relativeX);

% 避免浮点误差导致asin输入超出[-1,1]
if sinPitch > single(1.0)
    sinPitch = single(1.0);
elseif sinPitch < single(-1.0)
    sinPitch = single(-1.0);
end

pitch = asin(sinPitch);

%% 四元数转Yaw

sinYaw = single(2.0) * ...
    (relativeW*relativeZ + relativeX*relativeY);

cosYaw = single(1.0) - single(2.0) * ...
    (relativeY*relativeY + relativeZ*relativeZ);

yaw = atan2(sinYaw, cosYaw);

%% 最终输出检查

if isfinite(roll) && ...
   isfinite(pitch) && ...
   isfinite(yaw) && ...
   zeroValid

    valid = true;
else

    roll  = single(0.0);
    pitch = single(0.0);
    yaw   = single(0.0);
    valid = false;
end

end

== matlab function Import_IMU/Balance_Target_XY ==
  data: simTime input; xLeftCmd output; enableControl input; imuValid input; xLeftActual input; yLeftActual input; xRightActual input; yRightActual input; roll input; pitch input; gyroX input; gyroY input; kpRoll input; kdRoll input; kpPitch input; kdPitch input; yLeftCmd output; xRightCmd output; yRightCmd output; deltaXPitch output; deltaYRoll output; controlState output; valid output
function [xLeftCmd, yLeftCmd, ...
          xRightCmd, yRightCmd, ...
          deltaXPitch, deltaYRoll, ...
          controlState, valid] = ...
    balance_target_xy( ...
    simTime, ...
    enableControl, imuValid, ...
    xLeftActual, yLeftActual, ...
    xRightActual, yRightActual, ...
    roll, pitch, gyroX, gyroY, ...
    kpRoll, kdRoll, ...
    kpPitch, kdPitch)
%#codegen
%
% 真实轮毂坐标目标生成器
%
% IMU坐标：
%   +X：向车头
%   +Y：从右侧指向左侧
%   +Z：向上
%
% 五连杆坐标：
%   +x：向车尾
%   +y：向下
%
% 输出：
%   xLeftCmd、yLeftCmd   左轮毂真实目标坐标
%   xRightCmd、yRightCmd 右轮毂真实目标坐标
%
% controlState:
%   0 = disabled
%   1 = moving to home while balancing
%   2 = home reached and balancing

persistent previousEnable
persistent startTime
persistent xLeftStart yLeftStart
persistent xRightStart yRightStart
persistent toleranceStartTime
persistent internalState

if isempty(previousEnable)
    previousEnable = false;

    startTime = 0.0;

    xLeftStart  = single(0.035);
    yLeftStart  = single(0.100);
    xRightStart = single(0.035);
    yRightStart = single(0.100);

    toleranceStartTime = -1.0;
    internalState = uint8(0);
end

%% 固定参数

xHome = single(0.035);
yHome = single(0.100);

homeTime = 5.0;          % 回Home时间，单位s
balanceRampTime = 1.0;   % 姿态修正增益渐入时间

positionTolerance = single(0.003);  % 3 mm
holdTime = 0.5;                   % 保持0.5 s

maxPitchShift = single(0.003);     % x方向最多修正±3 mm
maxRollDifference = single(0.3); % 左右总高度差最多±3 mm

%% 默认输出

xLeftCmd  = xLeftActual;
yLeftCmd  = yLeftActual;
xRightCmd = xRightActual;
yRightCmd = yRightActual;

deltaXPitch = single(0);
deltaYRoll  = single(0);

controlState = uint8(0);
valid = false;

%% 数据有效性检查

dataValid = ...
    isfinite(xLeftActual)  && ...
    isfinite(yLeftActual)  && ...
    isfinite(xRightActual) && ...
    isfinite(yRightActual) && ...
    isfinite(roll)         && ...
    isfinite(pitch)        && ...
    isfinite(gyroX)        && ...
    isfinite(gyroY);

if ~enableControl || ~imuValid || ~dataValid

    previousEnable = false;
    internalState = uint8(0);
    toleranceStartTime = -1.0;

    return;
end

%% 检测使能上升沿

if ~previousEnable

    startTime = simTime;

    % 记录使能瞬间的真实轮毂位置
    xLeftStart  = xLeftActual;
    yLeftStart  = yLeftActual;

    xRightStart = xRightActual;
    yRightStart = yRightActual;

    toleranceStartTime = -1.0;

    internalState = uint8(1);
end

previousEnable = true;

%% 计算回Home平滑系数

uHome = (simTime - startTime) / homeTime;

if uHome < 0.0
    uHome = 0.0;
elseif uHome > 1.0
    uHome = 1.0;
end

% 半余弦平滑，起点和终点速度均为零
homeBlend = single(0.5 - 0.5*cos(pi*uHome));

%% 左右腿基础轨迹：当前位置平滑移动到Home

xLeftBase = ...
    xLeftStart + ...
    homeBlend * (xHome - xLeftStart);

yLeftBase = ...
    yLeftStart + ...
    homeBlend * (yHome - yLeftStart);

xRightBase = ...
    xRightStart + ...
    homeBlend * (xHome - xRightStart);

yRightBase = ...
    yRightStart + ...
    homeBlend * (yHome - yRightStart);

%% 姿态修正渐入系数

uBalance = (simTime - startTime) / balanceRampTime;

if uBalance < 0.0
    uBalance = 0.0;
elseif uBalance > 1.0
    uBalance = 1.0;
end

balanceBlend = single(0.5 - 0.5*cos(pi*uBalance));

%% Roll修正
%
% 正Roll：
% 左侧较高、右侧较低。
%
% 修正：
% 左腿缩短，右腿伸长。

deltaYRoll = balanceBlend * ...
    (kpRoll * roll + kdRoll * gyroX);

%% Pitch修正
%
% IMU +X向车头；
% 腿部+x向车尾；
% 因此使用负号。

deltaXPitch = -balanceBlend * ...
    (kpPitch * pitch + kdPitch * gyroY);

%% 修正限幅

if deltaYRoll > maxRollDifference
    deltaYRoll = maxRollDifference;
elseif deltaYRoll < -maxRollDifference
    deltaYRoll = -maxRollDifference;
end

if deltaXPitch > maxPitchShift
    deltaXPitch = maxPitchShift;
elseif deltaXPitch < -maxPitchShift
    deltaXPitch = -maxPitchShift;
end

%% 最终左右轮毂目标坐标

% Pitch：左右轮毂同时前后移动
xLeftCmd  = xLeftBase  + deltaXPitch;
xRightCmd = xRightBase + deltaXPitch;

% Roll：左右轮毂产生高度差
yLeftCmd  = yLeftBase  - single(0.5) * deltaYRoll;
yRightCmd = yRightBase + single(0.5) * deltaYRoll;

%% 判断是否进入稳定平衡状态

if uHome >= 1.0

    errorLeft = sqrt( ...
        (xLeftActual - xLeftCmd)^2 + ...
        (yLeftActual - yLeftCmd)^2);

    errorRight = sqrt( ...
        (xRightActual - xRightCmd)^2 + ...
        (yRightActual - yRightCmd)^2);

    if errorLeft <= positionTolerance && ...
       errorRight <= positionTolerance

        if toleranceStartTime < 0.0
            toleranceStartTime = simTime;
        end

        if simTime - toleranceStartTime >= holdTime
            internalState = uint8(2);
        end

    else
        toleranceStartTime = -1.0;
    end
end

controlState = internalState;
valid = true;

end

== matlab function Import_IMU/FiveBar_IK_Left ==
  data: xCmd input; alphaCmd output; yCmd input; alphaActual input; betaActual input; L1 input; L2 input; L3 input; L4 input; L5 input; betaCmd output; valid output
function [alphaCmd, betaCmd, valid] = fivebar_ik( ...
    xCmd, yCmd, ...
    alphaActual, betaActual, ...
    L1, L2, L3, L4, L5)
%#codegen
%
% Five-Bar Inverse Kinematics
% 五连杆逆运动学
%
% 功能：
% 已知轮毂中心目标坐标(xCmd,yCmd)，
% 求两个主动关节目标角alphaCmd、betaCmd。
%
% 坐标定义：
%
% Alpha电机中心：
%   O = (0,0)
%
% Beta电机中心：
%   D = (L5,0)
%
% 腿部局部坐标：
%   +x：Alpha电机指向Beta电机
%   +y：竖直向下
%
% 连杆：
%   O-A = L1
%   A-B = L2
%   D-C = L4
%   C-B = L3
%
% 输入：
%   xCmd        轮毂目标x，单位m
%   yCmd        轮毂目标y，单位m
%   alphaActual 当前实际Alpha关节角，单位rad
%   betaActual  当前实际Beta关节角，单位rad
%   L1~L5       五连杆尺寸，单位m
%
% 输出：
%   alphaCmd    Alpha关节目标角，单位rad
%   betaCmd     Beta关节目标角，单位rad
%   valid       目标位置是否可达
%
% 解选择方法：
% 每个主动关节都会产生两个候选解，
% 本函数选择最接近当前实际关节角的解，
% 避免机构突然跳到另一种装配构型。

%% 默认输出

alphaCmd = alphaActual;
betaCmd  = betaActual;
valid    = false;

%% 检查输入是否有效

inputValid = ...
    isfinite(xCmd)        && ...
    isfinite(yCmd)        && ...
    isfinite(alphaActual) && ...
    isfinite(betaActual)  && ...
    isfinite(L1)          && ...
    isfinite(L2)          && ...
    isfinite(L3)          && ...
    isfinite(L4)          && ...
    isfinite(L5);

if ~inputValid
    return;
end

if L1 <= single(0) || ...
   L2 <= single(0) || ...
   L3 <= single(0) || ...
   L4 <= single(0) || ...
   L5 <= single(0)

    return;
end

%% =========================================================
%  求Alpha侧两个候选解
%
%  Alpha电机中心O = (0,0)
%  主动杆长度L1
%  被动杆长度L2
% ==========================================================

dxAlpha = xCmd;
dyAlpha = yCmd;

rAlphaSquared = ...
    dxAlpha * dxAlpha + ...
    dyAlpha * dyAlpha;

rAlpha = sqrt(rAlphaSquared);

% 检查目标是否在Alpha侧二连杆工作空间内
if rAlpha < single(1.0e-6)
    return;
end

if rAlpha > L1 + L2
    return;
end

if rAlpha < abs(L1 - L2)
    return;
end

% 从余弦定理求主动杆与目标连线之间的夹角
cosDeltaAlpha = ...
    (L1 * L1 + rAlphaSquared - L2 * L2) / ...
    (single(2) * L1 * rAlpha);

% 处理浮点数误差
tolerance = single(1.0e-5);

if cosDeltaAlpha > single(1) + tolerance || ...
   cosDeltaAlpha < single(-1) - tolerance

    return;
end

if cosDeltaAlpha > single(1)
    cosDeltaAlpha = single(1);
elseif cosDeltaAlpha < single(-1)
    cosDeltaAlpha = single(-1);
end

phiAlpha = atan2(dyAlpha, dxAlpha);
deltaAlpha = acos(cosDeltaAlpha);

% Alpha两个候选角
alphaCandidate1 = phiAlpha + deltaAlpha;
alphaCandidate2 = phiAlpha - deltaAlpha;

%% =========================================================
%  求Beta侧两个候选解
%
%  Beta电机中心D = (L5,0)
%  主动杆长度L4
%  被动杆长度L3
% ==========================================================

dxBeta = xCmd - L5;
dyBeta = yCmd;

rBetaSquared = ...
    dxBeta * dxBeta + ...
    dyBeta * dyBeta;

rBeta = sqrt(rBetaSquared);

% 检查目标是否在Beta侧二连杆工作空间内
if rBeta < single(1.0e-6)
    return;
end

if rBeta > L4 + L3
    return;
end

if rBeta < abs(L4 - L3)
    return;
end

cosDeltaBeta = ...
    (L4 * L4 + rBetaSquared - L3 * L3) / ...
    (single(2) * L4 * rBeta);

if cosDeltaBeta > single(1) + tolerance || ...
   cosDeltaBeta < single(-1) - tolerance

    return;
end

if cosDeltaBeta > single(1)
    cosDeltaBeta = single(1);
elseif cosDeltaBeta < single(-1)
    cosDeltaBeta = single(-1);
end

phiBeta = atan2(dyBeta, dxBeta);
deltaBeta = acos(cosDeltaBeta);

% Beta两个候选角
betaCandidate1 = phiBeta + deltaBeta;
betaCandidate2 = phiBeta - deltaBeta;

%% =========================================================
%  将候选角转换到当前实际关节角附近
%
%  例如：
%  当前角为3.2 rad，
%  候选角为-3.0 rad，
%  实际上二者可能只相差约0.08 rad。
% ==========================================================

alphaCandidate1 = alphaActual + ...
    wrap_to_pi_single(alphaCandidate1 - alphaActual);

alphaCandidate2 = alphaActual + ...
    wrap_to_pi_single(alphaCandidate2 - alphaActual);

betaCandidate1 = betaActual + ...
    wrap_to_pi_single(betaCandidate1 - betaActual);

betaCandidate2 = betaActual + ...
    wrap_to_pi_single(betaCandidate2 - betaActual);

%% 选择距离当前实际角最近的Alpha解

alphaError1 = abs(alphaCandidate1 - alphaActual);
alphaError2 = abs(alphaCandidate2 - alphaActual);

if alphaError1 <= alphaError2
    alphaCmd = alphaCandidate1;
else
    alphaCmd = alphaCandidate2;
end

%% 选择距离当前实际角最近的Beta解

betaError1 = abs(betaCandidate1 - betaActual);
betaError2 = abs(betaCandidate2 - betaActual);

if betaError1 <= betaError2
    betaCmd = betaCandidate1;
else
    betaCmd = betaCandidate2;
end

%% 最终有效性检查

if ~isfinite(alphaCmd) || ~isfinite(betaCmd)
    alphaCmd = alphaActual;
    betaCmd  = betaActual;
    return;
end

valid = true;

end


function angleWrapped = wrap_to_pi_single(angle)
% 将角度限制到[-pi,pi)

piSingle = single(pi);
twoPi = single(2) * piSingle;

angleWrapped = mod(angle + piSingle, twoPi) - piSingle;

end
